simulink model "superhet"  (R2015b)
settings: Solver=VariableStepAuto  StartTime=0.0  StopTime=10.0  RelTol=1e-3
libraries: rfmathmodels1 x4, simrfV2elements x2, powerlib_meascontrol x1, elec_lib x1
settings Model: Creator=dominikguz  LastModifiedBy=dominikguz

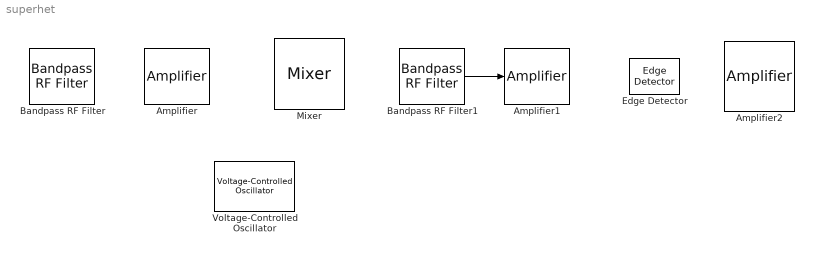
== system superhet ==
  Amplifier : rfmathmodels1/Amplifier  model_select=Linear  linGaindB=0  GindB=0  iip3=30  am2pm=10  PwrAMPMStart=10  PwrAMPMEnd=inf  amam=[2.1587 1.1517]  ampm=[4.0033 9.1040]  x=[8.1081 1.5413 6.5202 -0.0718]  y=[4.6645 2.0965 10.88 -0.003]  p=0.5  GoutdB=0  vsat=1  method_select=Noise factor  ntemp=290  nfigure=3.01  nfactor=2  seed=67987
  Amplifier1 : rfmathmodels1/Amplifier  model_select=Linear  linGaindB=0  GindB=0  iip3=30  am2pm=10  PwrAMPMStart=10  PwrAMPMEnd=inf  amam=[2.1587 1.1517]  ampm=[4.0033 9.1040]  x=[8.1081 1.5413 6.5202 -0.0718]  y=[4.6645 2.0965 10.88 -0.003]  p=0.5  GoutdB=0  vsat=1  method_select=Noise factor  ntemp=290  nfigure=3.01  nfactor=2  seed=67987
  Amplifier2 : simrfV2elements/Amplifier  classname=amplifier  DataSource=Data file  File=simrfV2_unitygain.s2p  Paramtype=S-parameters  Sparam=[0 0;1 0]  SparamFreq=1e9 Hz  SparamZ0=50  Residues=0  Poles=0  DF={0 0; 1 0}  Source_linear_gain=Available power gain  linear_gain=0 dB  Zin=50  Zout=50  Source_Poly=Even and odd order  Poly_Coeffs=[0 1]  IPType=Output  IP2=inf dBm  IP3=inf dBm  P1dB=inf dBm  Psat=inf dBm  Gcomp=inf dBm  NF=0  InternalGrounding=on  SourceFreq=Extracted from data source  PlotFreq=[1e9:1e6:3e9] Hz  PlotType=X-Y plane  YParam1=S11  YFormat1=Magnitude (decibels)  YParam2=None  YFormat2=Magnitude (decibels)  YOption=Linear  XOption=Linear  SparamRepresentation=Time domain (rationalfit)  FitTol=-40  FitOpt=Fit individually  AutoImpulseLength=on  ImpulseLength=1e-10 s
  Bandpass RF Filter : rfmathmodels1/Bandpass RF Filter  method=Butterworth  filttype=Bandpass  N=3  flo=1.9998e9  fhi=2.0002e9  Rp=1  Rs=10  MaxLength=32  Fc=2e9  Ts=1e-6
  Bandpass RF Filter1 : rfmathmodels1/Bandpass RF Filter  method=Butterworth  filttype=Bandpass  N=3  flo=1.9998e9  fhi=2.0002e9  Rp=1  Rs=10  MaxLength=32  Fc=2e9  Ts=1e-6
  Edge Detector : powerlib_meascontrol/Logic/Edge Detector  model=Rising  ic=0  Ts=0
  Mixer : simrfV2elements/Mixer  classname=mixer  Source_linear_gain=Available power gain  linear_gain=0 dB  Zin=50  Zout=50  ZLO=inf  Source_Poly=Even and odd order  Poly_Coeffs=[0 1]  IPType=Output  IP2=Inf dBm  IP3=Inf dBm  P1dB=Inf dBm  Psat=Inf dBm  Gcomp=Inf dBm  NF=0  InternalGrounding=on
  Voltage-Controlled Oscillator : elec_lib/Integrated Circuits/Voltage-Controlled Oscillator  tabulated=0  f_nom=1000 Hz  v_nom=0.5 V  df_dv=0 Hz/V  v_min=0 V  v_max=1 V  v_vec=[ 0 0.2 0.4 0.6 0.8 1 ] V  f_vec=[-1000 -329 -51 162 342 500] Hz  v_out=1 V  r_in=Inf Ohm  r_out=0 Ohm  model_dynamics=0  time_constant=0.001 s  f_ini=1000 Hz
  wires:
  Bandpass RF Filter1/1 -> Amplifier1/1
